simulink model "pH2"  (R2023a)
settings: Solver=VariableStepAuto  StartTime=0.0  StopTime=10.0  RelTol=1e-3
settings Model: Creator=meghn  LastModifiedBy=meghn

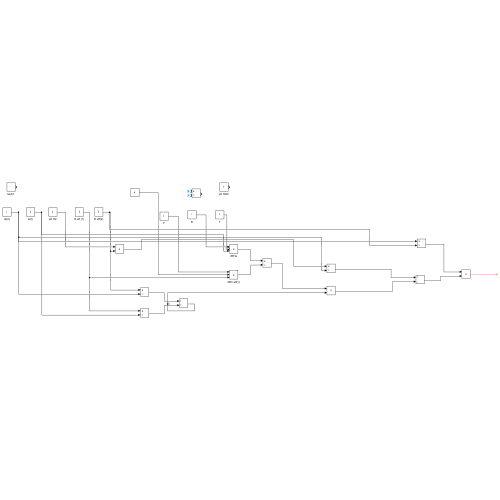
[thumbnail: Simulink's stored preview of the top-level diagram]
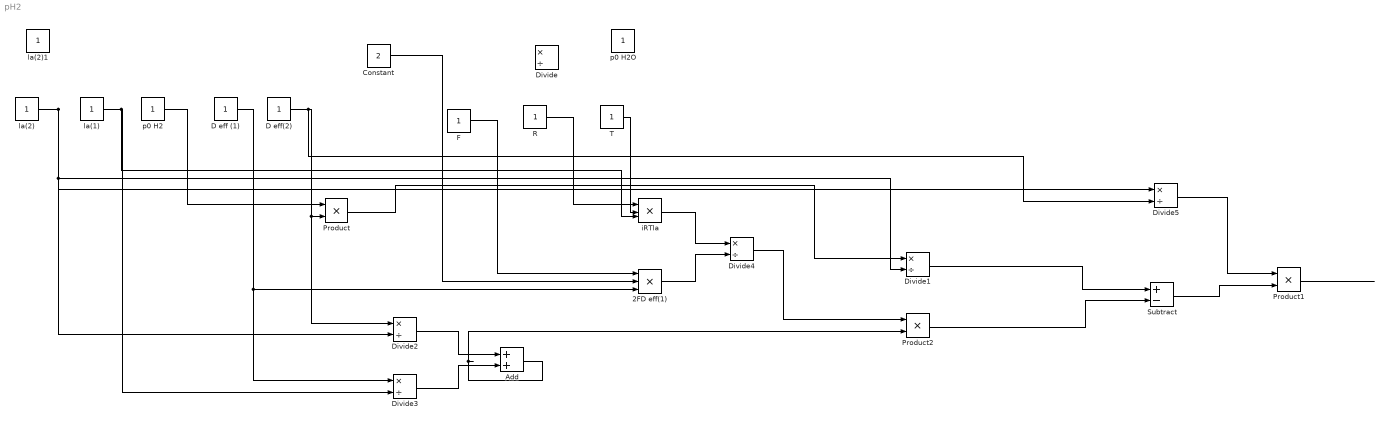
== system pH2 ==
  2FD eff(1) : Product  Inputs=3  RndMeth=Round
  Add : Sum
  Constant : Constant  Value=2
  D eff (1) : Constant
  D eff(2) : Constant
  Divide{,1..5} (6 alike) : Product  Inputs=*/
  F : Constant
  Product : Product
  Product1 : Product
  Product2 : Product
  R : Constant
  Subtract : Sum  Inputs=+-
  T : Constant
  iRTla : Product  Inputs=4
  la(1) : Constant
  la(2) : Constant
  la(2)1 : Constant
  p0 H2 : Constant
  p0 H2O : Constant
  wires:
  p0 H2/1 -> Product/1
  D eff(2)/1 -> Divide5/2, Divide2/1, Product/2
  Product/1 -> Divide1/1
  la(2)/1 -> Divide5/1, Divide2/2, Divide1/2
  D eff (1)/1 -> 2FD eff(1)/3, Divide3/1
  la(1)/1 -> iRTla/4, Divide3/2
  Divide2/1 -> Add/1
  Divide3/1 -> Add/2
  Add/1 -> Product2/2
  R/1 -> iRTla/1
  T/1 -> iRTla/3
  F/1 -> 2FD eff(1)/1
  Constant/1 -> 2FD eff(1)/2
  iRTla/1 -> Divide4/1
  2FD eff(1)/1 -> Divide4/2
  Divide4/1 -> Product2/1
  Divide1/1 -> Subtract/1
  Product2/1 -> Subtract/2
  Subtract/1 -> Product1/2
  Divide5/1 -> Product1/1
  Product1/1 -> ?
